simulink model "FluxMapID_ref"  (R2022b)
settings: Solver=FixedStepDiscrete  StartTime=0.0  StopTime=160  FixedStep=0.000005  RelTol=1e-3  EnableMultiTasking=on
settings Model: RequirementInfo={} %GIDa_fe9045fd_0412_4b6e_8206_617cc20e6fde  FPTRunName=Active  Creator=ts  LastModifiedBy=hufnagelde
settings SolverCC: AlgebraicLoopSolver=TrustRegion  PositivePriorityOrder=on  AutoInsertRateTranBlk=on
settings DataIOCC: SaveOutput=off  SignalLogging=off  DSMLogging=off  SaveTime=off
settings OptimizationCC: DefaultParameterBehavior=Inlined  UseDivisionForNetSlopeComputation=on  GainParamInheritBuiltInType=on  UseFloatMulNetSlope=on  DefaultUnderspecifiedDataType=single  UseSpecifiedMinMax=on  InlineInvariantSignals=on  PassReuseOutputArgsAs=Individual arguments  ZeroExternalMemoryAtStartup=off  ZeroInternalMemoryAtStartup=off  NoFixptDivByZeroProtection=on  EfficientFloat2IntCast=on  LifeSpan=1  MaxStackSize=64  OptimizeBlockOrder=speed  DifferentSizesBufferReuse=on  EfficientTunableParamExpr=on
settings DebuggingCC: UnconnectedInputMsg=warning  UnconnectedOutputMsg=warning  UnconnectedLineMsg=warning  BusObjectLabelMismatch=error  AllowSymbolicDim=off  SFUnexpectedBacktrackingDiag=warning  SFNoUnconditionalDefaultTransitionDiag=warning  SFExecutionAtInitializationDiag=none  SFMachineParentedDataDiag=warning  ArithmeticOperatorsInVariantConditions=warning
settings HardwareCC: ProdBitPerPointer=32  ProdBitPerSizeT=32  ProdBitPerPtrDiffT=32  ProdLargestAtomicInteger=Long  ProdLargestAtomicFloat=Double  ProdWordSize=32  ProdLongLongMode=on  ProdHWDeviceType=ARM Compatible->ARM Cortex-R  HardwareBoardFeatureSet=SoCBlockset
settings ModelReferenceCC: EnableRefExpFcnMdlSchedulingChecks=on
settings SFSimCC: SimGenImportedTypeDefs=on  MATLABDynamicMemAlloc=off
settings RTWCC: Description=Embedded Coder  SystemTargetFile=ert.tlc  GenCodeOnly=on  TemplateMakefile=ert_default_tmf  GenerateReport=on  BuildConfiguration=Faster Runs  IncludeHyperlinkInReport=on  LaunchReport=on  GenerateTraceInfo=on  GenerateTraceReport=on  GenerateTraceReportSl=on  GenerateTraceReportSf=on  GenerateTraceReportEml=on  GenerateCodeMetricsReport=on  CheckMdlBeforeBuild=Warning  DLArmComputeVersion=19.05
settings CodeAppCC: ForceParamTrailComments=on  IgnoreCustomStorageClasses=off  OperatorAnnotations=on  SimulinkDataObjDesc=on  SFDataObjDesc=on  MATLABFcnDesc=on  CustomSymbolStrGlobalVar=rt$M$R$N  CustomSymbolStrType=$N$M$R_t  CustomSymbolStrFcn=$N$M$F  CustomSymbolStrMacro=$N$M  InsertBlockDesc=on  StateflowObjectComments=on  MATLABSourceComments=on  EnableCustomComments=on  ReqsInCode=on
settings ERTTargetCC: TargetLangStandard=C99 (ISO)  CodeReplacementLibrary=GNU C99 extensions  MultiwordLength=2048  IncludeMdlTerminateFcn=off  CombineSignalStateStructs=on  SuppressErrorStatus=on  IncludeFileDelimiter=UseQuote  SupportAbsoluteTime=off  CodeInterfacePackaging=Reusable function  SupportNonFinite=off  RemoveResetFunc=off  InlinedParameterPlacement=NonHierarchical  MultiInstanceErrorCode=Warning  RootIOFormat=Part of model data structure  ERTCustomFileTemplate=example_file_process.tlc  GlobalDataDefinition=InSourceFile  GlobalDataReference=InSourceFile  ERTFilePackagingFormat=CompactWithDataFile  SuppressUnreachableDefaultCases=off
settings ConfigComp: CovScope=ReferencedModels  CovSaveName=covdata_rollAP  CovMetricSettings=dcmtrwe  CovHTMLOptions=-sRT=1 -aTS=1 -bRG=1 -bTC=1 -hTR=1 -nFC=0 -scm=1 -bcm=1 -xEv=0  CovSaveCumulativeToWorkspaceVar=on  CovSaveSingleToWorkspaceVar=on  CovCumulativeVarName=covCumulativeData_rollAP  CovReportOnPause=off  CovExternalEMLEnable=off  CovSFcnEnable=off

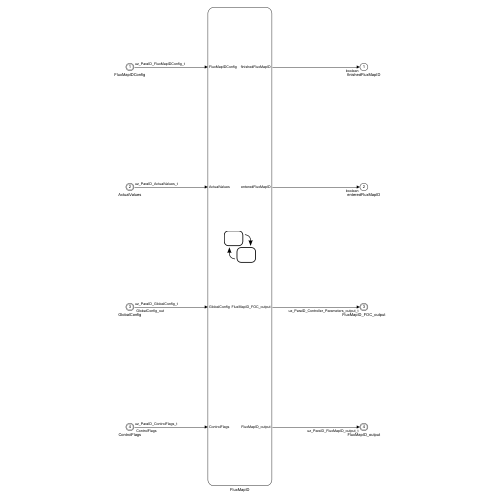
[thumbnail: Simulink's stored preview of the top-level diagram]
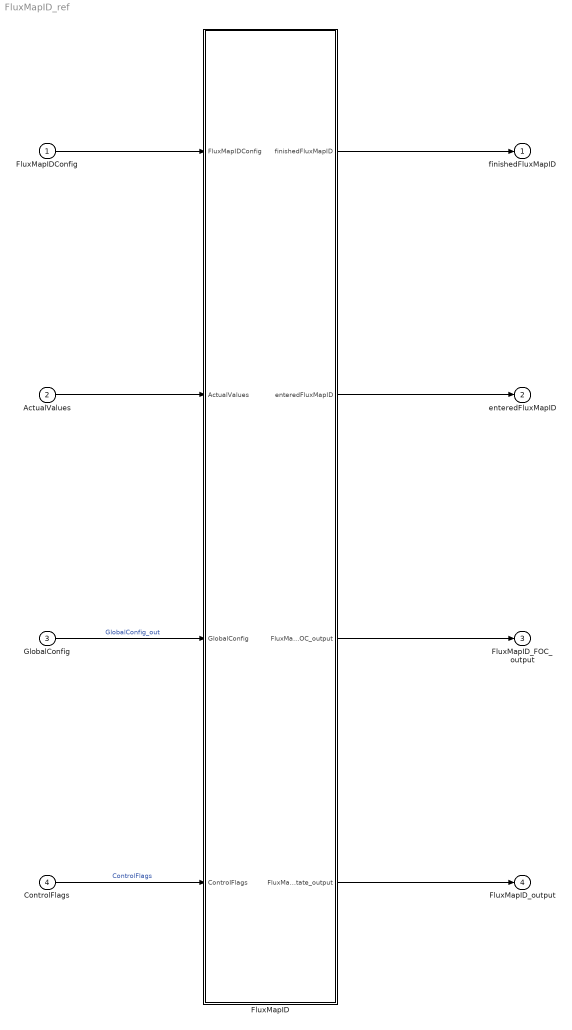
== system FluxMapID_ref ==
  FluxMapIDConfig : Inport  OutDataTypeStr=Bus: uz_ParaID_FluxMapIDConfig_t  PortDimensions=1  SampleTime=[5.0000000000000002e-05,0]  BusOutputAsStruct=on
  ActualValues : Inport  Port=2  OutDataTypeStr=Bus: uz_ParaID_ActualValues_t  PortDimensions=1  SampleTime=[5.0000000000000002e-05,0]  BusOutputAsStruct=on
  GlobalConfig : Inport  Port=3  OutDataTypeStr=Bus: uz_ParaID_GlobalConfig_t  PortDimensions=1  SampleTime=[5.0000000000000002e-05,0]  BusOutputAsStruct=on
  ControlFlags : Inport  Port=4  OutDataTypeStr=Bus: uz_ParaID_ControlFlags_t  PortDimensions=1  SampleTime=[5.0000000000000002e-05,0]  BusOutputAsStruct=on
  FluxMapID : Stateflow chart  TreatAsAtomicUnit=on
  finishedFluxMapID : Outport  OutDataTypeStr=boolean  PortDimensions=1  SampleTime=[5.0000000000000002e-05,0]
  enteredFluxMapID : Outport  Port=2  OutDataTypeStr=boolean  PortDimensions=1  SampleTime=[5.0000000000000002e-05,0]
  FluxMapID_FOC_output : Outport  Port=3  OutDataTypeStr=Bus: uz_ParaID_Controller_Parameters_output_t  PortDimensions=1  SampleTime=[5.0000000000000002e-05,0]  BusOutputAsStruct=on
  FluxMapID_output : Outport  Port=4  OutDataTypeStr=Bus: uz_ParaID_FluxMapID_output_t  PortDimensions=1  SampleTime=[5.0000000000000002e-05,0]  BusOutputAsStruct=on
  wires:
  FluxMapIDConfig/1 -> FluxMapID/1(FluxMapIDConfig)
  ActualValues/1 -> FluxMapID/2(ActualValues)
  GlobalConfig/1 -> FluxMapID/3(GlobalConfig)  "GlobalConfig_out"
  ControlFlags/1 -> FluxMapID/4(ControlFlags)  "ControlFlags"
  FluxMapID/1(finishedFluxMapID) -> finishedFluxMapID/1
  FluxMapID/2(enteredFluxMapID) -> enteredFluxMapID/1
  FluxMapID/3(FluxMapID_FOC_output) -> FluxMapID_FOC_output/1
  FluxMapID/4(FluxMapID_state_output) -> FluxMapID_output/1

== stateflow chart FluxMapID_ref/FluxMapID ==
  settings: updateMethod=DISCRETE  sampleTime=1/d_f_states
  note: Flux Map identification
  state AMMstate
    entry:
    initParams;
    enteredFluxMapID = boolean(1);
    FluxMapID_FOC_output.enableFOC_current=boolean(1);
    FluxMapID_FOC_output.activeState = uint16(400);
    if(FluxMapIDConfig.IDstepsize==0)
    IDstepsize_loc = single(1.0);
    end
    if(FluxMapIDConfig.IQstepsize==0)
    IQstepsize_loc = single(1.0);
    end
    during:
    if(FluxMapIDConfig.start_FM_ID==1)
    FluxMapID_FOC_output.i_dq_ref.d=i_d_R_online+i_d_ref_AMM;
    FluxMapID_FOC_output.i_dq_ref.q=i_q_ref_AMM;
    if(FluxMapIDConfig.identR == 1)
    if(FluxMapID_FOC_output.activeState ~= 403)
    FluxMapID_state_output.R_s = identRes;
    end
    if(FluxMapIDConfig.R_s_ref ~= 0.0 && FluxMapIDConfig.Temp_ref ~= 0.0)
    FluxMapID_state_output.WindingTemp = ((FluxMapID_state_output.R_s/FluxMapIDConfig.R_s_ref)-1)....
    *254.453+FluxMapIDConfig.Temp_ref;
    end
    end
    if(FluxMapIDConfig.identR == 0)
    i_d_R_online = single(0.0);
    FluxMapID_state_output.WindingTemp= single(65);
    end
    else
    FluxMapID_FOC_output.i_dq_ref.d=single(0);
    FluxMapID_FOC_output.i_dq_ref.q=single(0);
    end
    exit:
    counter = uint32(1);
    AMMcounter = uint32(0);
    AMMn = uint32(0);
    AMMj = uint32(0);
    repetitionCounter = uint32(0);
    i_q_ref_AMM = single(0.0);
    i_d_ref_AMM = single(0.0);
    state initAMM
      entry:
      FluxMapID_FOC_output.activeState = uint16(401);
      repetitionCounter = uint32(0);
      NumberOfIDpoints = uint32(abs(FluxMapIDConfig.IDstop-FluxMapIDConfig.IDstart)/IDstepsize_loc+1);
      NumberOfIQpoints = uint32(abs(FluxMapIDConfig.IQstop-FluxMapIDConfig.IQstart)/IQstepsize_loc+1);
      NumberOfPoints = uint32(NumberOfIDpoints*NumberOfIQpoints);
    state AMMheating
      entry:
      FluxMapID_FOC_output.activeState = uint16(420);
      i_q_ref_AMM = single(FluxMapIDConfig.IQstop);
      i_d_ref_AMM = single(FluxMapIDConfig.IDstart);
      exit:
      i_d_ref_AMM = i_d_ref_AMM_loc;
      i_q_ref_AMM = i_q_ref_AMM_loc;
    state AMMnewRef
      entry:
      counter_time = uint32(1);
      FluxMapID_FOC_output.activeState = uint16(402);
      if((FluxMapIDConfig.IDstart + single(AMMn) * IDstepsize_loc) <= FluxMapIDConfig.IDstop)
      i_d_ref_AMM = single(FluxMapIDConfig.IDstart + single(AMMn) * IDstepsize_loc);
      if(mod(single(AMMn),((abs(FluxMapIDConfig.IDstop-FluxMapIDConfig.IDstart))/IDstepsize_loc)+1) == 0)
      if((FluxMapIDConfig.IQstart + single(AMMj) * IQstepsize_loc) <= FluxMapIDConfig.IQstop)
      i_q_ref_AMM = single(FluxMapIDConfig.IQstart + single(AMMj) * IQstepsize_loc);
      AMMj = AMMj + 1;
      else
      i_q_ref_AMM = single(0.0);
      i_d_ref_AMM = single(0.0);
      end
      end
      end
      during: counter_time = counter_time +1;
    state AMMcooling
      entry:
      FluxMapID_FOC_output.activeState = uint16(410);
      i_q_ref_AMM = single(0.0);
      i_d_ref_AMM = single(0.0);
      exit:
      i_d_ref_AMM = i_d_ref_AMM_loc;
      i_q_ref_AMM = i_q_ref_AMM_loc;
    state AMMcompleted
      entry:
      counter_time = uint32(1);
      FluxMapID_FOC_output.activeState = uint16(450);
      AMMcounter = uint32(0);
      AMMn = uint32(0);
      AMMj = uint32(0);
      repetitionCounter = uint32(0);
      i_q_ref_AMM = single(0.0);
      i_d_ref_AMM = single(0.0);
      during:
      counter_time = counter_time +1;
      FluxMapID_FOC_output.resetIntegrator=boolean(1);
      exit:
      finishedFluxMapID=boolean(1);
      enteredFluxMapID = boolean(0);
      reset_FOC_output
    state whatsNext
      entry:
      i_d_ref_AMM_loc = i_d_ref_AMM;
      i_q_ref_AMM_loc = i_q_ref_AMM;
    state AMMcollectData
      entry: counter_time = uint32(1);
      FluxMapID_FOC_output.activeState = uint16(403);
      repetitionCounter = repetitionCounter + 1;
      i_d_R_online = single(0.0);
      if(AMMn >= (NumberOfIDpoints-1))
      AMMn = uint32(0);
      else
      AMMn = AMMn + 1;
      end
      FluxMapID_state_output.external_Measurement_Flag=boolean(1);
      during: counter_time = counter_time +1;
      exit:
      FluxMapID_state_output.external_Measurement_Flag=boolean(0);
    state waitForCollectToFinish
      entry:
      counter_time = uint32(1);
      FluxMapID_FOC_output.activeState = uint16(404);
      during:
      counter_time = counter_time +1;
      exit:
    (default) -> initAMM
    initAMM -> AMMheating [order 2] : [FluxMapID_state_output.WindingTemp < 60 && ....
        | FluxMapIDConfig.start_FM_ID==1]
    whatsNext -> AMMheating [order 3] : [FluxMapID_state_output.WindingTemp < 60]
    initAMM -> AMMcooling [order 1] : [FluxMapID_state_output.WindingTemp > 70 && ....
        | FluxMapIDConfig.start_FM_ID==1]
    initAMM -> AMMnewRef [order 3] : [FluxMapID_state_output.WindingTemp >=60 && ....
        | FluxMapID_state_output.WindingTemp <=70 && ....
        | FluxMapIDConfig.start_FM_ID==1]
    AMMheating -> AMMnewRef : [FluxMapID_state_output.WindingTemp >= 60]
    AMMcooling -> AMMnewRef : [FluxMapID_state_output.WindingTemp <= 60]
    whatsNext -> AMMcooling [order 2] : [FluxMapID_state_output.WindingTemp > 70]
    whatsNext -> AMMnewRef [order 4] : [FluxMapID_state_output.WindingTemp >=60 && FluxMapID_state_output.WindingTemp <= 70]
    AMMnewRef -> AMMcollectData : [three_sec_transition_counter == counter_time]
    whatsNext -> AMMcompleted [order 1] : [repetitionCounter >= NumberOfPoints]
    waitForCollectToFinish -> whatsNext : [three_sec_transition_counter == counter_time]
    AMMcollectData -> waitForCollectToFinish : [collection_transition_counter == counter_time]
  state Waiting
    entry:
    %wait for activation of
    %FluxMapID
    %donothing
  note: ---
  Waiting -> AMMstate [order 1] : [ControlFlags.startFluxMapID==1 && ....
      | GlobalConfig.Reset==0 && GlobalConfig.ACCEPT==1]
  (default) -> Waiting
  Waiting -> Waiting [order 2] : [GlobalConfig.Reset==1]{finishedFluxMapID=boolean(0);
      | enteredFluxMapID=boolean(0);initParams;}
  AMMstate -> Waiting : [GlobalConfig.Reset==1 || GlobalConfig.FluxMapID==0....
      | || GlobalConfig.enableParameterID==0]
      | {enteredFluxMapID=boolean(0); initParams;}
  AMMcompleted -> Waiting : [one_sec_transition_counter == counter_time]
  data: fun function_output; FluxMapIDConfig input Bus: uz_ParaID_FluxMapIDConfig_t; counter local; vd2_counter local; finishedFluxMapID output boolean; enteredFluxMapID output boolean; AMMcounter local; AMMj local; AMMn local; i_d_ref_AMM local; i_d_ref_AMM_loc local; i_q_ref_AMM local; i_q_ref_AMM_loc local; NumberOfIDpoints local; NumberOfIQpoints local; NumberOfPoints local; i_d_R_online local; repetitionCounter local; id2_counter local; FluxMapID_FOC_output output Bus: uz_ParaID_Controller_Parameters_output_t; ActualValues input Bus: uz_ParaID_ActualValues_t; GlobalConfig input Bus: uz_ParaID_GlobalConfig_t; ControlFlags input Bus: uz_ParaID_ControlFlags_t; FluxMapID_state_output output Bus: uz_ParaID_FluxMapID_output_t; vd1_counter local; id1_counter local; R_s_array local single size=50; IQstepsize_loc local single; IDstepsize_loc local single; three_sec_transition_counter local uint32; one_sec_transition_counter local uint32; collection_transition_counter local; counter_time local
  function fun = identRes:
    | function fun = identRes 
    | 
    | 	if(counter <= uint32(0.2/GlobalConfig.sampleTimeISR))%meas
    |         i_d_R_online = single(-FluxMapIDConfig.identRAmp);
    |             if(counter >= uint32(0.1/GlobalConfig.sampleTimeISR) && counter < uint32(0.2/GlobalConfig.sampleTimeISR))
    |                 vd1_counter = vd1_counter + ActualValues.v_dq.d;
    |                 id1_counter = id1_counter + ActualValues.i_dq.d;
    |             end
    | 	end
    |         
    | 	if(counter > uint32(0.2/GlobalConfig.sampleTimeISR) && counter <= uint32(0.4/GlobalConfig.sampleTimeISR))
    |         i_d_R_online = single(FluxMapIDConfig.identRAmp);
    |             if(counter >= uint32(0.3/GlobalConfig.sampleTimeISR) && counter < uint32(0.4/GlobalConfig.sampleTimeISR))
    |                 vd2_counter = vd2_counter + ActualValues.v_dq.d;
    |                 id2_counter = id2_counter + ActualValues.i_dq.d;
    |             end
    | 	end
    |         
    | 	if(counter == uint32(0.4/GlobalConfig.sampleTimeISR + 1) )
    |         i_d_R_online = single(-FluxMapIDConfig.identRAmp);
    |         vd1_counter=vd1_counter/(0.1/GlobalConfig.sampleTimeISR);
    |         id1_counter=id1_counter/(0.1/GlobalConfig.sampleTimeISR);
    |         vd2_counter=vd2_counter/(0.1/GlobalConfig.sampleTimeISR);
    |         id2_counter=id2_counter/(0.1/GlobalConfig.sampleTimeISR);
    |         R_s_array(1,1) = single((vd2_counter-vd1_counter)/(id2_counter-id1_counter));
    |         RefreshDataRegister;
    |         FluxMapID_state_output.R_s = mean(R_s_array);
    |         counter = uint32(1);
    | 	end
    |         
    | counter = counter + 1;
    | fun = single(FluxMapID_state_output.R_s);
    | end
  function RefreshDataRegister:
    | function RefreshDataRegister
    | 
    | m=length(R_s_array);
    |     for k= uint16(0):uint16(m-2)
    |         R_s_array(m-k)=R_s_array(m-(k+1));
    |     end
    | 
    | end
  function initParams:
    | function initParams
    | 
    | %This is used instead of "after(1.0,sec) to ensure the same transition time
    | %independelty of the sampletime in the c-code
    | one_sec_transition_counter = uint32(1/GlobalConfig.sampleTimeISR);
    | three_sec_transition_counter = uint32(3/GlobalConfig.sampleTimeISR);
    | collection_transition_counter = uint32(FluxMapIDConfig.AMMsampleTime/GlobalConfig.sampleTimeISR);
    | % initialize variables
    | vd1_counter 		= single(0.0);
    | id1_counter        	= single(0.0);
    | vd2_counter 		= single(0.0);
    | id2_counter        	= single(0.0);
    | i_d_R_online        = single(0.0);
    | i_d_ref_AMM_loc     = single(0.0);
    | i_q_ref_AMM_loc     = single(0.0);
    | R_s_array           = single(zeros(50,1));
    | counter_time        = uint32(0); 
    | counter = uint32(1);
    | AMMcounter = uint32(0);
    | AMMn = uint32(0);
    | AMMj = uint32(0);
    | repetitionCounter = uint32(0);
    | i_q_ref_AMM = single(0.0);
    | i_d_ref_AMM = single(0.0);
    | IDstepsize_loc = single(FluxMapIDConfig.IDstepsize);
    | IQstepsize_loc = single(FluxMapIDConfig.IQstepsize);
    | %Outputs
    | FluxMapID_FOC_output.n_ref_FOC         	= single(0.0);
    | FluxMapID_FOC_output.M_ref_FOC        	= single(0.0);
    | FluxMapID_FOC_output.i_dq_ref.d      	= single(0.0);
    | FluxMapID_FOC_output.i_dq_ref.q       	= single(0.0);
    | FluxMapID_FOC_output.i_dq_ref.zero      = single(0.0);
    | FluxMapID_FOC_output.enableFOC_speed   	= boolean(0);
    | FluxMapID_FOC_output.enableFOC_current  = boolean(0);
    | FluxMapID_FOC_output.enableFOC_torque   = boolean(0);
    | FluxMapID_FOC_output.resetIntegrator 	= boolean(0);
    | FluxMapID_FOC_output.Kp_id_out          = single(GlobalConfig.Kp_id);
    | FluxMapID_FOC_output.Kp_iq_out         	= single(GlobalConfig.Kp_iq);
    | FluxMapID_FOC_output.Kp_n_out         	= single(GlobalConfig.Kp_n);
    | FluxMapID_FOC_output.Ki_id_out         	= single(GlobalConfig.Ki_id);
    | FluxMapID_FOC_output.Ki_iq_out        	= single(GlobalConfig.Ki_iq);
    | FluxMapID_FOC_output.Ki_n_out          	= single(GlobalConfig.Ki_n);
    | FluxMapID_FOC_output.activeState        = uint16(0);
    | finishedFluxMapID                       = boolean(0);
    | 
    | FluxMapID_state_output.R_s                    = single(FluxMapIDConfig.R_s_ref);
    | FluxMapID_state_output.WindingTemp            = single(FluxMapIDConfig.Temp_ref);
    | FluxMapID_state_output.external_Measurement_Flag = boolean(0);
    | end
  function reset_FOC_output:
    | function reset_FOC_output
    | %Outputs
    | FluxMapID_FOC_output.n_ref_FOC         	= single(0.0);
    | FluxMapID_FOC_output.M_ref_FOC        	= single(0.0);
    | FluxMapID_FOC_output.i_dq_ref.d      	= single(0.0);
    | FluxMapID_FOC_output.i_dq_ref.q       	= single(0.0);
    | FluxMapID_FOC_output.i_dq_ref.zero      = single(0.0);
    | FluxMapID_FOC_output.enableFOC_speed   	= boolean(0);
    | FluxMapID_FOC_output.enableFOC_current  = boolean(0);
    | FluxMapID_FOC_output.enableFOC_torque   = boolean(0);
    | FluxMapID_FOC_output.resetIntegrator 	= boolean(0);
    | FluxMapID_FOC_output.Kp_id_out          = single(GlobalConfig.Kp_id);
    | FluxMapID_FOC_output.Kp_iq_out         	= single(GlobalConfig.Kp_iq);
    | FluxMapID_FOC_output.Kp_n_out         	= single(GlobalConfig.Kp_n);
    | FluxMapID_FOC_output.Ki_id_out         	= single(GlobalConfig.Ki_id);
    | FluxMapID_FOC_output.Ki_iq_out        	= single(GlobalConfig.Ki_iq);
    | FluxMapID_FOC_output.Ki_n_out          	= single(GlobalConfig.Ki_n);
    | FluxMapID_FOC_output.activeState        = uint16(0);
    | end
